simulink model "StandardModel_tl"  (Simulink 6.4)
settings: Solver=FixedStepDiscrete  StartTime=0.0  StopTime=10.0  FixedStep=0.01  RelTol=1e-3
PreLoadFcn:
  | if exist('tl_preloadfcn','file'), tl_preloadfcn(gcs,95); end
PostLoadFcn:
  | if exist('tl_postloadfcn','file'), tl_postloadfcn(gcs,95); end
InitFcn:
  | if exist('tlds_start','file'), tlds_start(gcs); end
undefined symbols (not defined in the file or in its folder): built, constant, Constant, in, Product, Relay, Saturate, Switch, UnitDelay
libraries: tllib x22
PreSaveFcn:
  | if exist('tl_presavefcn','file'), tl_presavefcn(gcs); end
settings Model: LastModifiedBy=alexh  DS_PROJECTFILE=StandardModel.dd  TL_MAIN_DATA=struct('date',733129.51061415509,'maxnumsimulations',10,'codeopt',struct('inliningthreshold',6,'target',['Generic ANSI-C'],'assembler',0,'optlevel',0,'linebreaklimit',100,'stateactcodinglimit',1,'functionsfor64bitops',1,'sections',1,'sfbitfields',1,'globalbitfields',0,'sharefunctions',0,'noinitstozero',0,'limidentlength',1,'decimals',1,'separatesearch',0,'cleancode',0,'optimizedbooltype',1,'keepsaturation',0,'extvarsharing',0,'outputstylefile','cconfig.xml','rootstylesheet','TL_CSourceCodeSS.xsl','addchecksum',0,'modelsaving',2,'browsecodegen',0),'frameopt',struct('exectime',1,'stacksize',1,'simconfig',['default EVM'],'targettimeout',1,'mexargs','-g','tcargs',''),'logopt',struct('plotinterval',0.1,'globalloggingmode',1),'export',struct('directory','.\export','sysfiles',1,'docfiles',0,'tools',0),'codecoveragelevel',0,'asapscript','asap2_all_in_one','docscript','tldoc_default','rtos',struct('enablemultirate',0,'currentrtos',['generic RTOS'],'autopriority',0,'autoinitalarm',1,'alarminitwithrestart',1,'alarmactivationkind',1,'alarmstartoffset',0),'advcodeopt',{{'ExtendedBlockComments','true','GenerateEmptyConditionalBranches','true','PolySpaceSupport','true','ScreenInfo','true'}})
settings DataIOCC: SaveFormat=StructureWithTime
settings DebuggingCC: StrictBusMsg=None

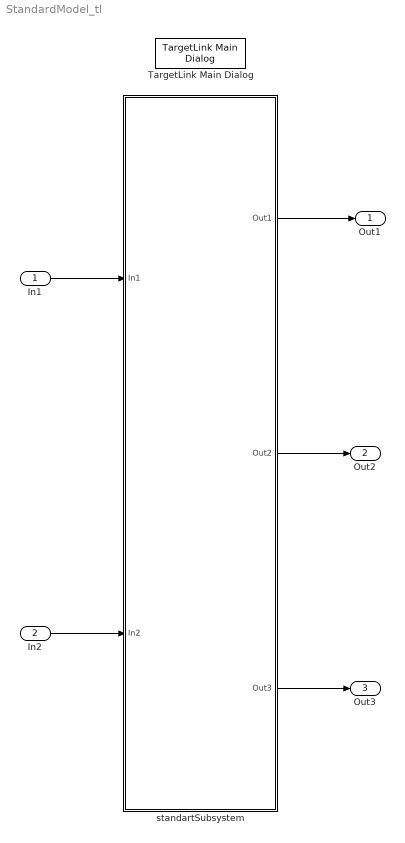
== system StandardModel_tl ==
  In1 : Inport
  In2 : Inport  Port=2
  TargetLink Main Dialog : tllib/TargetLink Main Dialog  SystemSampleTime=-1  flp_block=none
  standartSubsystem : Subsystem  Tag=TargetLink Simulation Frame
      settings: CopyFcn=if exist('tl_copyfcn','file'), tl_copyfcn(gcbh); end  NameChangeFcn=if exist('tl_framenamechangefcn','file'), tl_framenamechangefcn(gcbh); end  OpenFcn=if exist('open_tlsubsystem','file'), open_tlsubsystem(gcbh); end
      mask Type: TL_SimFrame
      mask Display: disp('TargetLink\nModel-\nin-the-loop\nmode')
  Out1 : Outport
  Out2 : Outport  Port=2
  Out3 : Outport  Port=3
  wires:
  In1/1 -> standartSubsystem/1(In1)
  In2/1 -> standartSubsystem/2(In2)
  standartSubsystem/1(Out1) -> Out1/1
  standartSubsystem/2(Out2) -> Out2/1
  standartSubsystem/3(Out3) -> Out3/1

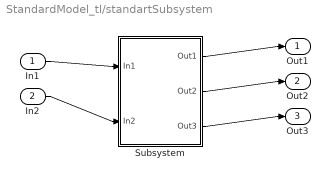
== system StandardModel_tl/standartSubsystem ==
  In1 : Inport  PortDimensions=1
  In2 : Inport  Port=2  PortDimensions=1
  Subsystem : Subsystem
      settings: OpenFcn=warndlg(get_param(gcb,'MaskHelp'),'Serious Warning');
      mask Type: TL_Enable
      mask Help: This subsystem keeps the TargetLink subsystem (subsystem with TargetLink blocks for production code generation), and is needed for the TargetLink simulation frame to work properly. DO NOT DELETE OR MODIFY IT!
  Out1 : Outport
  Out2 : Outport  Port=2
  Out3 : Outport  Port=3
  wires:
  In1/1 -> Subsystem/1(In1)
  In2/1 -> Subsystem/2(In2)
  Subsystem/1(Out1) -> Out1/1
  Subsystem/2(Out2) -> Out2/1
  Subsystem/3(Out3) -> Out3/1

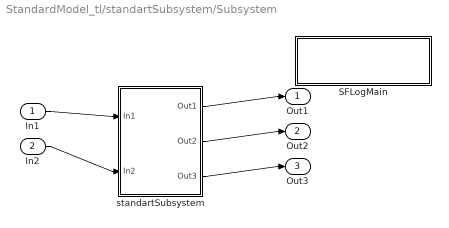
== system StandardModel_tl/standartSubsystem/Subsystem ==
  In1 : Inport  PortDimensions=1
  In2 : Inport  Port=2  PortDimensions=1
  SFLogMain : Subsystem
      mask Type: TL_StateflowLoggingMain
      mask Display:
      | plot([0 0 1 1 0 0 1 1 0],[0 1 1 0 0 0.05 0.05 0.95 0.95]);
      | disp('Stateflow Logging Main\nDO NOT DELETE')
  standartSubsystem : Subsystem  Tag=MIL Subsystem  Description=a
      settings: CopyFcn=if exist('tl_copyfcn','file'), tl_copyfcn(gcbh); end  NameChangeFcn=if exist('tl_namechangefcn','file'), tl_namechangefcn(gcbh); end  DestroyFcn=if exist('update_tl_main_dlg','file'), update_tl_main_dlg('TL_subs_display'); end
  Out1 : Outport
  Out2 : Outport  Port=2
  Out3 : Outport  Port=3
  wires:
  In1/1 -> standartSubsystem/1(In1)
  In2/1 -> standartSubsystem/2(In2)
  standartSubsystem/1(Out1) -> Out1/1
  standartSubsystem/2(Out2) -> Out2/1
  standartSubsystem/3(Out3) -> Out3/1

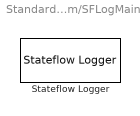
== system StandardModel_tl/standartSubsystem/Subsystem/SFLogMain ==
  Stateflow Logger : tllib/Extras/Stateflow Logger  data=struct('date',730486)  sflogparam=struct('charts',33,'sfblocks',{{'StandardModel_tl/standartSubsystem/Subsystem/standartSubsystem/AtomicSubsystem1/StateChart'}},'machines',32,'globallogopt',1,'modelname','StandardModel_tl','debugmodeactive',1)  flp_block=tldummylib/Stateflow Logger

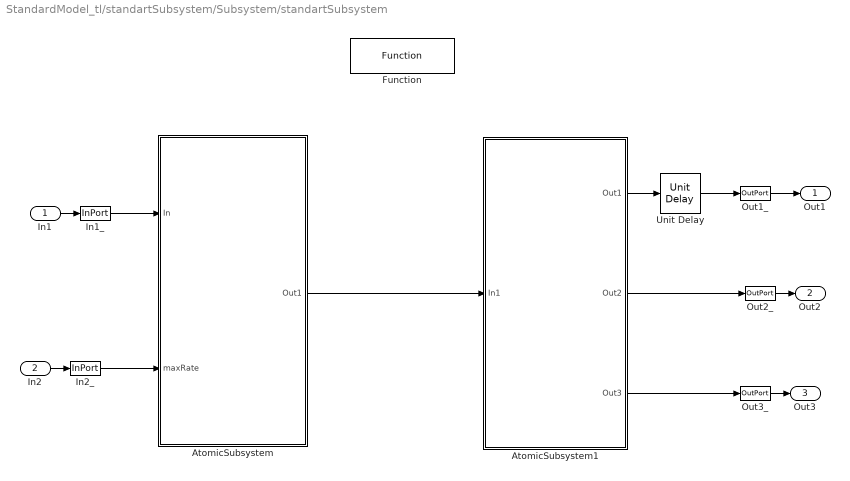
== system StandardModel_tl/standartSubsystem/Subsystem/standartSubsystem ==
  In1 : Inport  PortDimensions=1
      settings: CopyFcn=if exist('tl_check_ports','file'), tl_check_ports(gcbh); end  NameChangeFcn=if exist('tl_check_ports','file'), tl_check_ports(gcbh); end
  In2 : Inport  Port=2  PortDimensions=1
      settings: CopyFcn=if exist('tl_check_ports','file'), tl_check_ports(gcbh); end  NameChangeFcn=if exist('tl_check_ports','file'), tl_check_ports(gcbh); end
  AtomicSubsystem : Subsystem  TreatAsAtomicUnit=on
  AtomicSubsystem1 : Subsystem  TreatAsAtomicUnit=on
  Function : tllib/Function  SystemSampleTime=-1  data=struct('revisionNumber',9,'description','','stepfunctionname','$S_$B','stepfunctionclass','default','forcerestartfunction',0,'restartfunctionname','RESTART_$S_$B','restartfunctionclass','default','forceinitfunction',0,'initfunctionname','INIT_$S_$B','initfunctionclass','default','forcetermfunction',0,'termfunctionname','TERM_$S_$B','termfunctionclass','default','subsystemid','default','forcereuse',0,'linkfile',0,'functionarglist',{{}},'unscaledarguments',0,'scalingpropagation',{{}},'incrcodegen',0,'ownedmodules',{{}},'destination','','addtestframe',0,'simmode',1,'codecomment','','codefile','','codecoveragelevel',0,'date',733114.67812809)  flp_block=tldummylib/Function
  In1_ : tllib/InPort  SystemSampleTime=-1  data=struct('logdata',struct('maxnumvals',inf,'plotchannels',[],'loggingmode',3,'channels',1),'output',struct('variable','','description','','name','$S_$B','width',1,'address','','max',NaN,'min',NaN,'class','default','type','Int16','scaling','','lsb',1,'offset',0,'arb',0,'freeze',1,'unit','','autoscalingmode',1,'lowerheadroom',1,'upperheadroom',1,'headroomunit','bit','keepdatatype',1,'castoutput',0,'show',0),'message',struct('name','','component','','accessor',''),'virtual',1,'scalingvalid',0,'date',733114.678131354)  flp_block=none  slscaleparams={'ShowAdditionalParam','off','DataType','auto','OutDataType','sfix(16)','OutScaling','2^0','SampleTime','-1'}
  In2_ : tllib/InPort  SystemSampleTime=-1  data=struct('logdata',struct('maxnumvals',inf,'plotchannels',[],'loggingmode',3,'channels',1),'output',struct('variable','','description','','name','$S_$B','width',1,'address','','max',300,'min',-800,'class','default','type','Int16','scaling','','lsb',2^-2,'offset',-4,'arb',0,'freeze',1,'unit','','autoscalingmode',1,'lowerheadroom',1,'upperheadroom',1,'headroomunit','bit','keepdatatype',1,'castoutput',0,'show',0),'message',struct('name','','component','','accessor',''),'virtual',1,'scalingvalid',0,'date',733116.429755926)  flp_block=none  slscaleparams={'ShowAdditionalParam','off','DataType','auto','OutDataType','sfix(16)','OutScaling','2^0','SampleTime','-1'}
  Out1_ : tllib/OutPort  SystemSampleTime=-1  data=struct('comment',struct('text','','placement',1),'logdata',struct('maxnumvals',inf,'plotchannels',[],'loggingmode',3,'channels',1),'output',struct('variable','','description','','name','$S_$B','width',1,'address','','max',NaN,'min',NaN,'class','default','type','Int16','scaling','','lsb',2^-1,'offset',-3,'arb',0,'freeze',1,'unit','','autoscalingmode',1,'lowerheadroom',1,'upperheadroom',1,'headroomunit','bit','keepdatatype',1,'checkmin',1,'checkmax',1,'castoutput',0,'show',0),'message',struct('name','','component',''),'virtual',0,'scalingvalid',0,'date',733116.428905822)  flp_block=none
  Out2_ : tllib/OutPort  SystemSampleTime=-1  data=struct('comment',struct('text','','placement',1),'logdata',struct('maxnumvals',inf,'plotchannels',[],'loggingmode',3,'channels',1),'output',struct('variable','','description','','name','$S_$B','width',1,'address','','max',NaN,'min',NaN,'class','default','type','Int16','scaling','','lsb',1,'offset',0,'arb',0,'freeze',1,'unit','','autoscalingmode',1,'lowerheadroom',1,'upperheadroom',1,'headroomunit','bit','keepdatatype',1,'checkmin',0,'checkmax',0,'castoutput',0,'show',0),'message',struct('name','','component',''),'virtual',1,'scalingvalid',0,'date',733114.678132257)  flp_block=none
  Out3_ : tllib/OutPort  SystemSampleTime=-1  data=struct('comment',struct('text','','placement',1),'logdata',struct('maxnumvals',inf,'plotchannels',[],'loggingmode',3,'channels',1),'output',struct('variable','','description','','name','$S_$B','width',1,'address','','max',NaN,'min',NaN,'class','default','type','Int32','scaling','','lsb',1,'offset',0,'arb',0,'freeze',1,'unit','','autoscalingmode',1,'lowerheadroom',1,'upperheadroom',1,'headroomunit','bit','keepdatatype',1,'checkmin',0,'checkmax',0,'castoutput',0,'show',0),'message',struct('name','','component',''),'virtual',1,'scalingvalid',0,'date',733114.678132801)  flp_block=none
  Unit Delay : tllib/Unit Delay  SystemSampleTime=-1  data=struct('comment',struct('text','','placement',1),'logdata',struct('maxnumvals',inf,'plotchannels',[],'loggingmode',3,'channels',1),'output',struct('variable','','description','','name','$S_$B','width',1,'address','','max',NaN,'min',NaN,'class','default','type','Int16','scaling','','lsb',1,'offset',0,'arb',0,'freeze',1,'unit','','autoscalingmode',1,'lowerheadroom',1,'upperheadroom',1,'headroomunit','bit','keepdatatype',1,'checkmin',0,'checkmax',0,'castoutput',0,'show',0),'state',struct('variable','','description','','name','X_$S_$B','width',1,'address','','max',NaN,'min',NaN,'class','default','type','Int16','scaling','','lsb',1,'offset',0,'arb',0,'freeze',1,'unit','','initial','-2'),'dt','-1','scalingvalid',0,'date',733116.440309815)  dt=-1  X0=-2  flp_block=built-in/UnitDelay
  Out1 : Outport
      settings: CopyFcn=if exist('tl_check_ports','file'), tl_check_ports(gcbh); end  NameChangeFcn=if exist('tl_check_ports','file'), tl_check_ports(gcbh); end
  Out2 : Outport  Port=2
      settings: CopyFcn=if exist('tl_check_ports','file'), tl_check_ports(gcbh); end  NameChangeFcn=if exist('tl_check_ports','file'), tl_check_ports(gcbh); end
  Out3 : Outport  Port=3
      settings: CopyFcn=if exist('tl_check_ports','file'), tl_check_ports(gcbh); end  NameChangeFcn=if exist('tl_check_ports','file'), tl_check_ports(gcbh); end
  wires:
  AtomicSubsystem1/3(Out3) -> Out3_/1
  Out3_/1 -> Out3/1
  AtomicSubsystem1/2(Out2) -> Out2_/1
  Out2_/1 -> Out2/1
  Out1_/1 -> Out1/1
  In2_/1 -> AtomicSubsystem/2(maxRate)
  In2/1 -> In2_/1
  In1_/1 -> AtomicSubsystem/1(In)
  In1/1 -> In1_/1
  AtomicSubsystem/1(Out1) -> AtomicSubsystem1/1(In1)
  AtomicSubsystem1/1(Out1) -> Unit Delay/1
  Unit Delay/1 -> Out1_/1

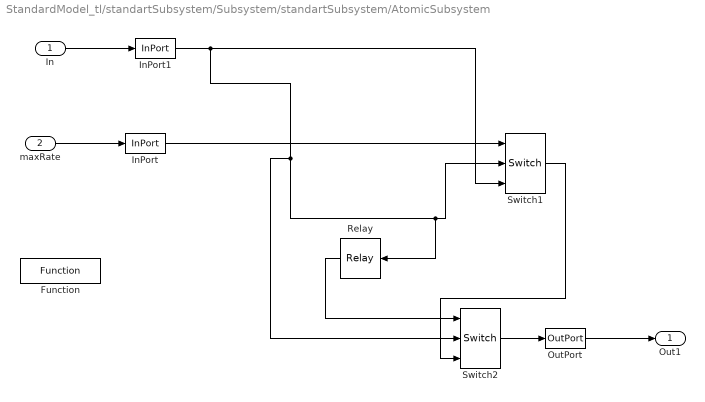
== system StandardModel_tl/standartSubsystem/Subsystem/standartSubsystem/AtomicSubsystem ==
  In : Inport
  maxRate : Inport  Port=2
  Function : tllib/Function  SystemSampleTime=-1  data=struct('revisionNumber',9,'description','','stepfunctionname','$S_$B','stepfunctionclass','STATIC_FCN','forcerestartfunction',0,'restartfunctionname','RESTART_$S_$B','restartfunctionclass','default','forceinitfunction',0,'initfunctionname','INIT_$S_$B','initfunctionclass','default','forcetermfunction',0,'termfunctionname','TERM_$S_$B','termfunctionclass','default','subsystemid','default','forcereuse',0,'linkfile',0,'functionarglist',{{}},'unscaledarguments',0,'scalingpropagation',{{}},'incrcodegen',0,'ownedmodules',{{}},'destination','','addtestframe',0,'simmode',1,'codecomment','','codefile','','codecoveragelevel',0)  flp_block=tldummylib/Function
  InPort : tllib/InPort  SystemSampleTime=-1  data=struct('logdata',struct('maxnumvals',inf,'plotchannels',[],'loggingmode',3,'channels',1),'output',struct('variable','','description','','name','$S_$B','width',1,'address','','max',NaN,'min',NaN,'class','FCN_REF_ARG','type','Int16','scaling','','lsb',1,'offset',0,'arb',0,'freeze',1,'unit','','autoscalingmode',1,'lowerheadroom',1,'upperheadroom',1,'headroomunit','bit','keepdatatype',1,'castoutput',0,'show',0),'message',struct('name','','component','','accessor',''),'virtual',1,'scalingvalid',0,'date',733116.436957025)  flp_block=none
  InPort1 : tllib/InPort  SystemSampleTime=-1  data=struct('logdata',struct('maxnumvals',inf,'plotchannels',[],'loggingmode',3,'channels',1),'output',struct('variable','','description','','name','$S_$B','width',1,'address','','max',NaN,'min',NaN,'class','FCN_ARG','type','Int16','scaling','','lsb',1,'offset',0,'arb',0,'freeze',1,'unit','','autoscalingmode',1,'lowerheadroom',1,'upperheadroom',1,'headroomunit','bit','keepdatatype',1,'castoutput',0,'show',0),'message',struct('name','','component','','accessor',''),'virtual',1,'scalingvalid',0,'date',733116.437838021)  flp_block=none
  OutPort : tllib/OutPort  SystemSampleTime=-1  data=struct('comment',struct('text','','placement',1),'logdata',struct('maxnumvals',inf,'plotchannels',[],'loggingmode',3,'channels',1),'output',struct('variable','','description','','name','$S_$B','width',1,'address','','max',NaN,'min',NaN,'class','FCN_RETURN','type','Int16','scaling','','lsb',1,'offset',0,'arb',0,'freeze',1,'unit','','autoscalingmode',1,'lowerheadroom',1,'upperheadroom',1,'headroomunit','bit','keepdatatype',1,'checkmin',0,'checkmax',0,'castoutput',0,'show',0),'message',struct('name','','component',''),'virtual',1,'scalingvalid',0,'date',733116.437082986)  flp_block=none
  Relay : tllib/Relay  Orientation=left  SystemSampleTime=-1  data=struct('comment',struct('text','','placement',1),'logdata',struct('maxnumvals',inf,'plotchannels',[],'loggingmode',3,'channels',1),'output',struct('variable','','description','','name','$S_$B','width',1,'address','','max',NaN,'min',NaN,'class','default','type','Int16','scaling','','lsb',1,'offset',0,'arb',0,'freeze',1,'unit','','autoscalingmode',1,'lowerheadroom',1,'upperheadroom',1,'headroomunit','bit','keepdatatype',1,'castoutput',0,'show',0),'onoutput',struct('variable','','description','','name','$S_$B_onoutput','width',1,'address','','max',NaN,'min',NaN,'class','CAL','type','Int16','scaling','','lsb',1,'offset',0,'arb',0,'freeze',1,'unit','','keepdatatype',1,'value','1'),'offoutput',struct('variable','','description','','name','$S_$B_offoutput','width',1,'address','','max',NaN,'min',NaN,'class','CAL','type','Int16','scaling','','lsb',1,'offset',0,'arb',0,'freeze',1,'unit','','keepdatatype',1,'value','0'),'onswitch',struct('variable','','description','','name','$S_$B_onswitch','width',1,'address','','max',NaN,'min',NaN,'class','CAL','type','Int16','scaling','','lsb',1,'offset',0,'arb',0,'freeze',1,'unit','','keepdatatype',1,'value','1','scalar',0),'offswitch',struct('variable','','description','','name','$S_$B_offswitch','width',1,'address','','max',NaN,'min',NaN,'class','CAL','type','Int16','scaling','','lsb',1,'offset',0,'arb',0,'freeze',1,'unit','','keepdatatype',1,'value','-1','scalar',0),'scalingvalid',0,'date',733110.704651296)  OnSwitchValue=1  OffSwitchValue=-1  OnOutputValue=1  OffOutputValue=0  flp_block=built-in/Relay  slscaleparams={'ShowAdditionalParam','off','OutputDataTypeScalingMode',['All ports same datatype'],'OutDataType','sfix(16)','OutScaling','2^0','ConRadixGroup',['Use specified scaling'],'SampleTime','-1'}
  Switch1 : tllib/Switch  SystemSampleTime=-1  data=struct('comment',struct('text','','placement',1),'logdata',struct('maxnumvals',inf,'plotchannels',[],'loggingmode',3,'channels',1),'output',struct('variable','','description','','name','$S_$B','width',1,'address','','max',NaN,'min',NaN,'class','default','type','Int16','scaling','','lsb',1,'offset',0,'arb',0,'freeze',1,'unit','','autoscalingmode',1,'lowerheadroom',1,'upperheadroom',1,'headroomunit','bit','keepdatatype',1,'checkmin',0,'checkmax',0,'castoutput',0,'show',0),'threshold',struct('variable','','description','','name','$S_$B_threshold','width',1,'address','','max',NaN,'min',NaN,'class','CAL','type','Int16','scaling','','lsb',1,'offset',0,'arb',0,'freeze',1,'unit','','keepdatatype',1,'value','0','scalar',0,'criteria',1),'scalingvalid',0,'date',733114.678123935)  threshold=0  flp_block=built-in/Switch  slscaleparams={'InputSameDT','on','ShowAdditionalParam','off','OutDataTypeMode',['Inherit via internal rule'],'RndMeth','Floor','SaturateOnIntegerOverflow','on','SampleTime','-1'}
  Switch2 : tllib/Switch  SystemSampleTime=-1  data=struct('comment',struct('text','','placement',1),'logdata',struct('maxnumvals',inf,'plotchannels',[],'loggingmode',3,'channels',1),'output',struct('variable','','description','','name','$S_$B','width',1,'address','','max',NaN,'min',NaN,'class','default','type','Int16','scaling','','lsb',1,'offset',0,'arb',0,'freeze',1,'unit','','autoscalingmode',1,'lowerheadroom',1,'upperheadroom',1,'headroomunit','bit','keepdatatype',1,'checkmin',0,'checkmax',0,'castoutput',0,'show',0),'threshold',struct('variable','','description','','name','$S_$B_threshold','width',1,'address','','max',NaN,'min',NaN,'class','CAL','type','Int16','scaling','','lsb',1,'offset',0,'arb',0,'freeze',1,'unit','','keepdatatype',1,'value','0','scalar',0,'criteria',1),'scalingvalid',0,'date',733114.678124653)  threshold=0  flp_block=built-in/Switch  slscaleparams={'InputSameDT','on','ShowAdditionalParam','off','OutDataTypeMode',['Inherit via internal rule'],'RndMeth','Floor','SaturateOnIntegerOverflow','on','SampleTime','-1'}
  Out1 : Outport
  wires:
  maxRate/1 -> InPort/1
  In/1 -> InPort1/1
  Relay/1 -> Switch2/1
  Switch1/1 -> Switch2/3
  Switch2/1 -> OutPort/1
  OutPort/1 -> Out1/1
  InPort/1 -> Switch1/1
  InPort1/1 -> Switch1/3, Switch1/2, Relay/1, Switch2/2

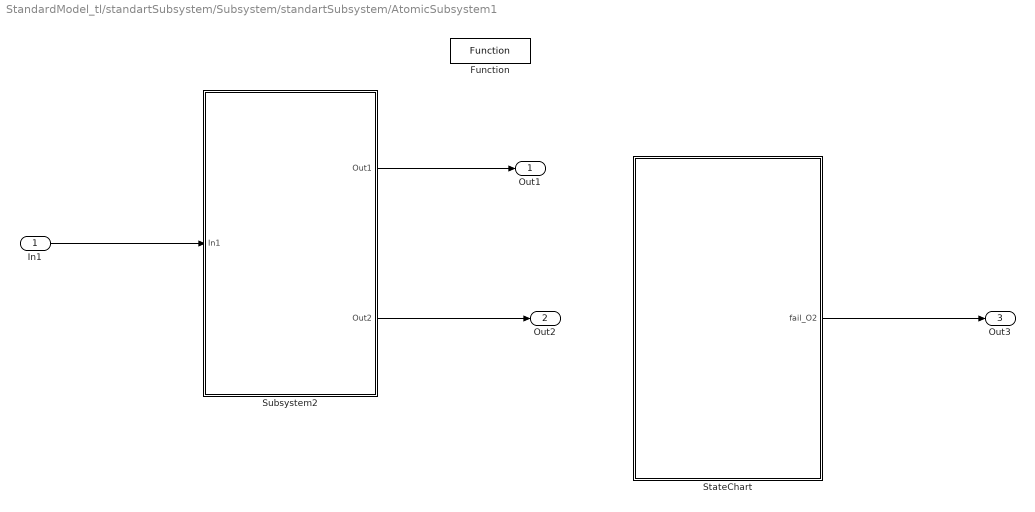
== system StandardModel_tl/standartSubsystem/Subsystem/standartSubsystem/AtomicSubsystem1 ==
  In1 : Inport
  Function : tllib/Function  SystemSampleTime=-1  data=struct('revisionNumber',9,'description','','stepfunctionname','$S_$B','stepfunctionclass','default','forcerestartfunction',0,'restartfunctionname','RESTART_$S_$B','restartfunctionclass','default','forceinitfunction',0,'initfunctionname','INIT_$S_$B','initfunctionclass','default','forcetermfunction',0,'termfunctionname','TERM_$S_$B','termfunctionclass','default','subsystemid','default','forcereuse',0,'linkfile',0,'functionarglist',{{}},'unscaledarguments',0,'scalingpropagation',{{}},'incrcodegen',0,'ownedmodules',{{}},'destination','','addtestframe',0,'simmode',1,'codecomment','','codefile','','codecoveragelevel',0,'date',733114.678125023)  flp_block=tldummylib/Function
  StateChart : Stateflow chart  Description=Stateflow diagram to determine control system operating mode
  Subsystem2 : Subsystem  TreatAsAtomicUnit=on
  Out1 : Outport
  Out2 : Outport  Port=2
  Out3 : Outport  Port=3
  wires:
  Subsystem2/2(Out2) -> Out2/1
  In1/1 -> Subsystem2/1(In1)
  Subsystem2/1(Out1) -> Out1/1
  StateChart/1(fail_O2) -> Out3/1

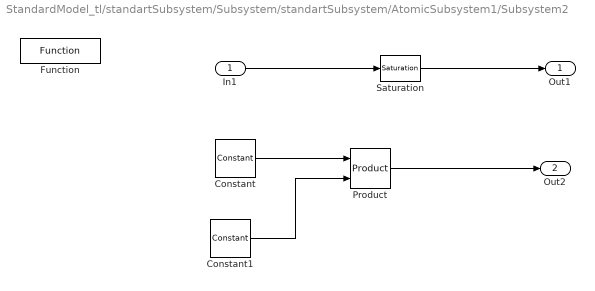
== system StandardModel_tl/standartSubsystem/Subsystem/standartSubsystem/AtomicSubsystem1/Subsystem2 ==
  In1 : Inport
  Constant : tllib/Constant  Value=constant  OutDataType=sfix(16)  ConRadixGroup=Use specified scaling  OutScaling=2^0  data=struct('comment',struct('text','','placement',1),'output',struct('variable','','description','','name','$S_$B','width',1,'address','','max',NaN,'min',NaN,'class','GLOBAL','type','Int16','scaling','','lsb',1,'offset',0,'arb',0,'freeze',1,'unit','','keepdatatype',1,'value','10','tolerance',1,'show',0),'dt','inf','scalingvalid',0,'date',733116.443451736)  constant=10  dt=inf  flp_block=built-in/Constant  slscaleparams={'VectorParams1D','on','ShowAdditionalParam','off','OutDataTypeMode',['Inherit from ''Constant value'''],'OutDataType','sfix(16)','OutScaling','2^0','ConRadixGroup',['Use specified scaling'],'SampleTime','inf'}
  Constant1 : tllib/Constant  Value=constant  OutDataType=sfix(16)  ConRadixGroup=Use specified scaling  OutScaling=2^0  data=struct('comment',struct('text','','placement',1),'output',struct('variable','','description','','name','$S_$B','width',1,'address','','max',NaN,'min',NaN,'class','CAL','type','Int16','scaling','','lsb',1,'offset',0,'arb',0,'freeze',1,'unit','','keepdatatype',1,'value','1','tolerance',1,'show',0),'dt','inf','scalingvalid',0,'date',733114.678125567)  constant=1  dt=inf  flp_block=built-in/Constant  slscaleparams={'VectorParams1D','on','ShowAdditionalParam','off','OutDataTypeMode',['Inherit from ''Constant value'''],'OutDataType','sfix(16)','OutScaling','2^0','ConRadixGroup',['Use specified scaling'],'SampleTime','inf'}
  Function : tllib/Function  SystemSampleTime=-1  data=struct('revisionNumber',9,'description','','stepfunctionname','$S_$B','stepfunctionclass','default','forcerestartfunction',0,'restartfunctionname','RESTART_$S_$B','restartfunctionclass','default','forceinitfunction',0,'initfunctionname','INIT_$S_$B','initfunctionclass','default','forcetermfunction',0,'termfunctionname','TERM_$S_$B','termfunctionclass','default','subsystemid','default','forcereuse',0,'linkfile',0,'functionarglist',{{}},'unscaledarguments',0,'scalingpropagation',{{}},'incrcodegen',0,'ownedmodules',{{}},'destination','','addtestframe',0,'simmode',1,'codecomment','','codefile','','codecoveragelevel',0,'date',733114.678126285)  flp_block=tldummylib/Function
  Product : tllib/Product  data=struct('comment',struct('text','','placement',1),'logdata',struct('maxnumvals',inf,'plotchannels',[],'loggingmode',3,'channels',1),'output',struct('variable','','description','','name','$S_$B','width',1,'address','','max',NaN,'min',NaN,'class','default','type','Int16','scaling','','lsb',1,'offset',0,'arb',0,'freeze',1,'unit','','autoscalingmode',1,'lowerheadroom',1,'upperheadroom',1,'headroomunit','bit','keepdatatype',1,'checkmin',0,'checkmax',0,'castoutput',0,'show',0),'inputs','*/','exceptionhandling',1,'scalingvalid',0,'date',733116.444770463)  flp_block=built-in/Product
  Saturation : tllib/Saturation  data=struct('comment',struct('text','','placement',1),'logdata',struct('maxnumvals',inf,'plotchannels',[],'loggingmode',3,'channels',1),'output',struct('variable','','description','','name','$S_$B','width',1,'address','','max',255,'min',0,'class','default','type','uint16','scaling','','lsb',1,'offset',0,'arb',0,'freeze',1,'unit','','autoscalingmode',1,'lowerheadroom',1,'upperheadroom',1,'headroomunit','bit','keepdatatype',1,'castoutput',0,'show',0),'lowerlimit',struct('variable','','description','','name','$S_$B_lower','width',1,'address','','max',NaN,'min',NaN,'class','CAL','type','Int16','scaling','','lsb',1,'offset',0,'arb',0,'freeze',1,'unit','','keepdatatype',1,'value','0','scalar',0),'upperlimit',struct('variable','','description','','name','$S_$B_upper','width',1,'address','','max',NaN,'min',NaN,'class','CAL','type','Int16','scaling','','lsb',1,'offset',0,'arb',0,'freeze',1,'unit','','keepdatatype',1,'value','2','scalar',0),'scalingvalid',0,'date',733114.678127731)  lower_limit=0  upper_limit=2  flp_block=built-in/Saturate  slscaleparams={'SampleTime','-1'}
  Out1 : Outport
  Out2 : Outport  Port=2
  wires:
  In1/1 -> Saturation/1
  Saturation/1 -> Out1/1
  Constant1/1 -> Product/2
  Constant/1 -> Product/1
  Product/1 -> Out2/1

== stateflow chart standartSubsystem/Subsystem/standartSubsystem/AtomicSubsystem1/StateChart ==
  settings: updateMethod=DISCRETE  sampleTime=0.01  description=$TL$ functionname=$O; $TL$
  state OxygenSensMode [parallel]
    settings: executionOrder=1
    settings: description=|
        | This state determines the validity of the exhaust gas oxygen sensor (EGO) data.
        | $TL$ name=$C_X_$O$R; $TL$
    state O2_Normal
      entry: fail_O2 = 0;
      settings: description=|
          | Normal EGO sensor operation gives a reliable indication of excess oxygen in the exhaust gas, from which air/fuel mixture can be inferred.
          | $TL$ name=$C_X_$O$R; $TL$
    state O2_Fail
      entry: fail_O2 = 1;
      settings: description=|
          | The EGO sensor has failed.
          | $TL$ name=$C_X_$O$R; $TL$
    state O2_Warmup
      entry: fail_O2 = 1;
      settings: description=|
          | The EGO sensor must come up to temperature before its data is reliable.
          | $TL$ name=$C_X_$O$R; $TL$
    O2_Warmup -> O2_Normal : [Calvariable== 5]
      settings: description=It is assumed that the time o2_t_thresh is sufficient for the sensor to warm up to operational temperature.
    (default) -> O2_Warmup
    O2_Normal -> O2_Fail : [Calvariable == 7]
      settings: description=The failure condition is indicated by excessive output voltage.
  data: Calvariable parameter int32 [0..1] =1; fail_O2 output int32 [0..1]
  data Calvariable settings: units=bar (absolute)
  data Calvariable settings: description=|
      | minimum manifold pressure expected at zero speed
      | $TL$ name=$C_V_$O$R; type=UInt16; lsb=2^-15; class=CAL; $TL$
  data fail_O2 settings: description=|
      | failure of oxygene sensor
      | $TL$ name=$O; type=Bool; class=MERGEABLE_DISP; $TL$
